simulink model "model_data_mesuare"  (R2020a)
settings: Solver=daessc  StartTime=0.0  StopTime=20  RelTol=1e-3
settings Model: Creator=artem  LastModifiedBy=artem

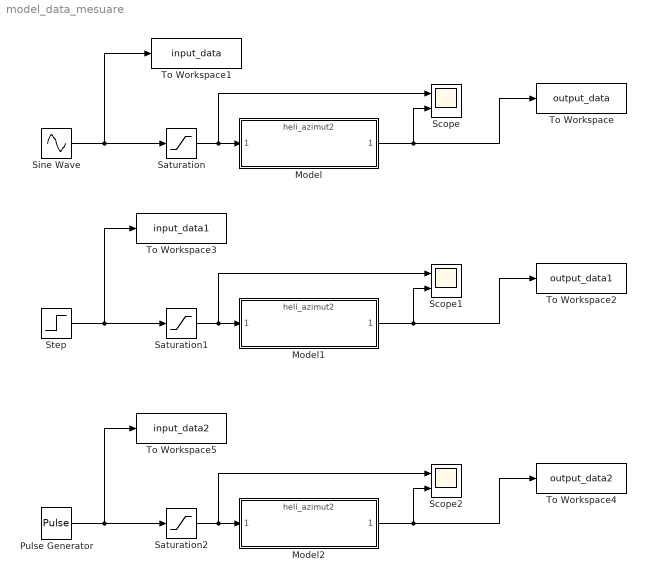
== system model_data_mesuare ==
  Model : ModelReference  ModelNameDialog=heli_azimut2.slxp  ModelReferenceVersion=1.106  CopyOfModelProtected=on
  Model1 : ModelReference  ModelNameDialog=heli_azimut2.slxp  ModelReferenceVersion=1.106  CopyOfModelProtected=on
  Model2 : ModelReference  ModelNameDialog=heli_azimut2.slxp  ModelReferenceVersion=1.106  CopyOfModelProtected=on
  Pulse Generator : DiscretePulseGenerator  PulseType=Time based  Amplitude=100  Period=5  PulseWidth=50
  Saturation : Saturate  UpperLimit=125  LowerLimit=-125
  Saturation1 : Saturate  UpperLimit=125  LowerLimit=-125
  Saturation2 : Saturate  UpperLimit=125  LowerLimit=-125
  Scope : Scope  NumInputPorts=2
  Scope1 : Scope  NumInputPorts=2
  Scope2 : Scope  NumInputPorts=2
  Sine Wave : Sin  Amplitude=50  SampleTime=0
  Step : Step  After=50  SampleTime=0
  To Workspace : ToWorkspace  VariableName=output_data  SaveFormat=Timeseries  SampleTime=-1
  To Workspace1 : ToWorkspace  VariableName=input_data  SaveFormat=Timeseries  SampleTime=-1
  To Workspace2 : ToWorkspace  VariableName=output_data1  SaveFormat=Timeseries  SampleTime=-1
  To Workspace3 : ToWorkspace  VariableName=input_data1  SaveFormat=Timeseries  SampleTime=-1
  To Workspace4 : ToWorkspace  VariableName=output_data2  SaveFormat=Timeseries  SampleTime=-1
  To Workspace5 : ToWorkspace  VariableName=input_data2  SaveFormat=Timeseries  SampleTime=-1
  wires:
  Saturation/1 -> Scope/1, Model/1
  Model/1 -> To Workspace/1, Scope/2
  Sine Wave/1 -> To Workspace1/1, Saturation/1
  Saturation1/1 -> Scope1/1, Model1/1
  Step/1 -> To Workspace3/1, Saturation1/1
  Model1/1 -> To Workspace2/1, Scope1/2
  Saturation2/1 -> Scope2/1, Model2/1
  Model2/1 -> To Workspace4/1, Scope2/2
  Pulse Generator/1 -> To Workspace5/1, Saturation2/1
